simulink model "Regelung_V3"  (R2021b)
settings: Solver=VariableStepAuto  StartTime=0.0  StopTime=10.0  RelTol=1e-3  EnableMultiTasking=on
values from neighbouring files (symbols this model uses):
  stPendel = block.DialogPrm(1).Data    [systemPendel_V3.m]
  x0 = block.DialogPrm(2).Data    [systemPendel_V3.m]
undefined symbols (not defined in the file or in its folder): K
settings Model: Creator=gong  LastModifiedBy=caio
settings SolverCC: AlgebraicLoopSolver=TrustRegion
settings DataIOCC: LimitDataPoints=on  SaveFormat=Array  ReturnWorkspaceOutputs=off
settings OptimizationCC: LifeSpan=inf
settings DebuggingCC: SFUnexpectedBacktrackingDiag=warning  SFNoUnconditionalDefaultTransitionDiag=warning  SFMachineParentedDataDiag=warning  ArithmeticOperatorsInVariantConditions=warning
settings HardwareCC: ProdBitPerPointer=32  ProdBitPerSizeT=32  ProdBitPerPtrDiffT=32  ProdLargestAtomicFloat=None  ProdIntDivRoundTo=Undefined  ProdEndianess=Unspecified  ProdWordSize=32  ProdHWDeviceType=32-bit Generic
settings ModelReferenceCC: PropagateSignalLabelsOutOfModel=off
settings SFSimCC: SimUseLocalCustomCode=off  CustomCodeUndefinedFunction=UseInterfaceOnly
settings RTWCC: RTWUseLocalCustomCode=off
settings CodeAppCC: StateflowObjectComments=on
settings GRTTargetCC: TargetLangStandard=C89/C90 (ANSI)
settings ConfigComp: CovMetricSettings=dw  CovSaveCumulativeToWorkspaceVar=on  CovSaveSingleToWorkspaceVar=on  CovExternalEMLEnable=off

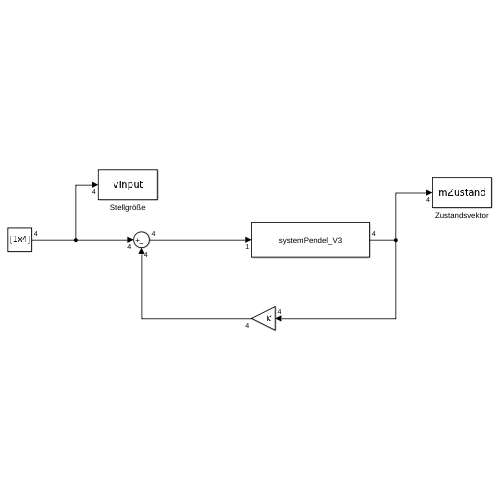
[thumbnail: Simulink's stored preview of the top-level diagram]
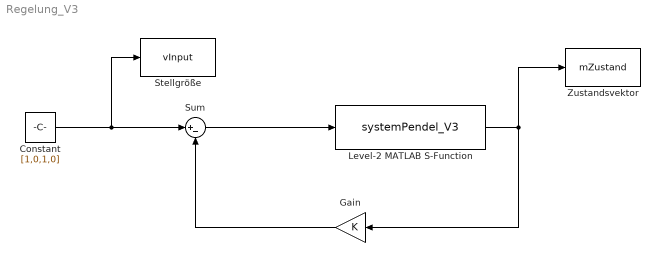
== system Regelung_V3 ==
  Constant : Constant  Value=[1,0,1,0]
  Gain : Gain  Gain=K
  Level-2 MATLAB S-Function : M-S-Function  FunctionName=systemPendel_V3  Parameters=stPendel,x0
  Stellgröße : ToWorkspace  VariableName=vInput  SaveFormat=Timeseries  SampleTime=-1
  Sum : Sum  Inputs=|+-
  Zustandsvektor : ToWorkspace  VariableName=mZustand  SaveFormat=Timeseries  SampleTime=-1
  wires:
  Level-2 MATLAB S-Function/1 -> Gain/1, Zustandsvektor/1
  Gain/1 -> Sum/2
  Constant/1 -> Stellgröße/1, Sum/1
  Sum/1 -> Level-2 MATLAB S-Function/1
